simulink model "ctrlSys"  (R2025b)
settings: Solver=ode14x  StartTime=0.0  StopTime=70  FixedStep=Ts_local  RelTol=1e-4
model workspace (MAT data in the model file):
  CtrlChoice = "GPC"
values from neighbouring files (symbols this model uses):
  Ts_ctrl = 0.1    [ctrlSys.sldd]
  u_b = 0.5864    [ctrlSys.sldd]
libraries: slpidlib x1
settings Model: DataDictionary=ctrlSys.sldd  SimulationMode=accelerator  Creator=LYG  LastModifiedBy=LYG
settings SolverCC: ZeroCrossControl=DisableAll

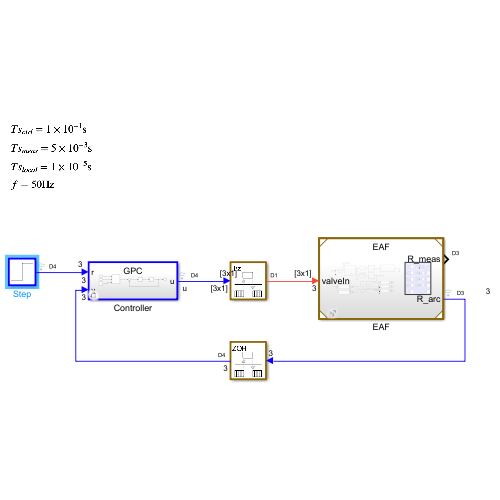
[thumbnail: Simulink's stored preview of the top-level diagram]
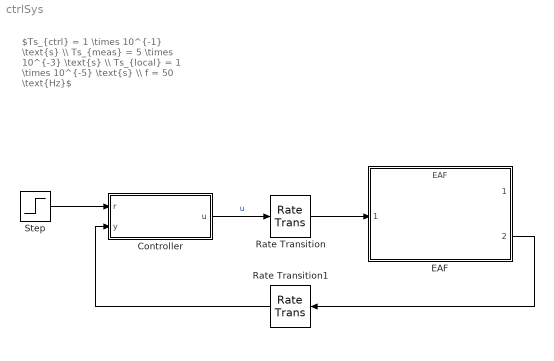
== system ctrlSys ==
  note: $Ts_{ctrl} = 1 \times 10^{-1} \text{s} \\ Ts_{meas} = 5 \times 10^{-3} \text{s} \\ Ts_{local} = 1 \times 10^{-5} \text{s} \\ f = 50 \text{Hz}$
  Controller : Subsystem  Variant=on
  EAF : ModelReference  ModelNameDialog=EAF.slx  SimulationMode=Normal  ModelReferenceVersion=1.75
  Rate Transition : RateTransition  InitialCondition=u_b  OutPortSampleTime=Ts_local
  Rate Transition1 : RateTransition  OutPortSampleTime=Ts_ctrl
  Step : Step  Time=20  Before=[0.025 0.01 0.075]  After=[0.025 0.02 0.075]  SampleTime=Ts_ctrl
  wires:
  Controller/1(u) -> Rate Transition/1  "u"
  Rate Transition/1 -> EAF/1
  EAF/2 -> Rate Transition1/1
  Step/1 -> Controller/1(r)
  Rate Transition1/1 -> Controller/2(y)

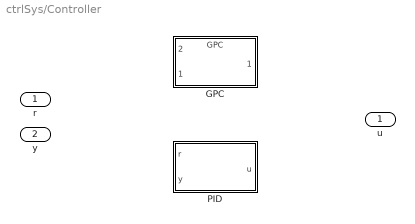
== system ctrlSys/Controller ==
  r : Inport
  y : Inport  Port=2
  GPC : ModelReference  ModelNameDialog=GPC.slx  SimulationMode=Normal  VariantControl="CtrlChoice == \"GPC\""  ModelReferenceVersion=1.202
      settings: PortSchema="{\"entries\":[{\"content\":{\"sides\":[{\"content\":{\"connectorIds\":[\"In2\",\"In1\"]},\"type\":\"ConnectorPlacement.EquallySpacedRectSide\",\"uuid\":\"c107f1c2-3547-45d9-8105-1f531098cad9\"},{\"content\":{\"connectorIds\":[\"Out1\"],\"side\":\"RIGHT\"},\"type\":\"ConnectorPlacement.EquallySpacedRectSide\",\"uuid\":\"edcbd001-1fd9-492d-b847-8c21cda39726\"},{\"content\":{\"side\":\"TOP\"},\"type\":\"ConnectorPlacement.EquallySpacedRectSide\",\"uuid\":\"231ba3de-6bd5-4532-a826-5d19b482de4e\"}]},\"type\":\"ConnectorPlacement.EquallySpacedConnector\",\"uuid\":\"eca704b6-0f9b-48e0-aad6-a98053cf6fe0\"}],\"packageUris\":[\"http://schema.mathworks.com/mf0/Connector/R2020b\"],\"version\":\"1.0\"}"
  PID : Subsystem  VariantControl="CtrlChoice == \"PID\""
  u : Outport

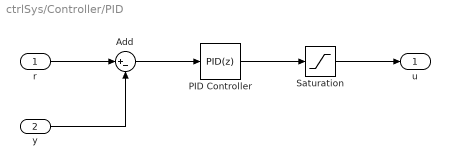
== system ctrlSys/Controller/PID ==
  r : Inport
  y : Inport  Port=2
  Add : Sum  Inputs=|+-
  PID Controller : slpidlib/PID Controller  Controller=PID  Form=Parallel  TimeDomain=Discrete-time  UseExternalTs=off  SampleTime=Ts_ctrl  IntegratorMethod=Forward Euler  FilterMethod=Forward Euler  ControllerParametersSource=internal  P=120  I=40  UseKiTs=off  D=0  UseExternalDerivativeSource=off  N=100  UseFilter=on  TunerSelectOption=Transfer Function Based (PID Tuner App)  InitialConditionSource=internal  InitialConditionForIntegrator=0  InitialConditionForFilter=0  DifferentiatorICPrevScaledInput=0  ExternalReset=none  TrackingMode=off  Kt=1  LimitOutput=off  SatLimitsSource=internal  UpperSaturationLimit=inf  LowerSaturationLimit=-inf  LinearizeAsGain=on  AntiWindupMode=none  Kb=1  LimitIntegrator=off  UpperIntegratorSaturationLimit=inf  LowerIntegratorSaturationLimit=-inf  POutMin=[]  POutMax=[]  IOutMin=[]  IOutMax=[]  DOutMin=[]  DOutMax=[]  NOutMin=[]  NOutMax=[]  SumOutMin=[]  SumOutMax=[]  SaturationOutMin=[]  SaturationOutMax=[]  PParamMin=[]  PParamMax=[]  IParamMin=[]  IParamMax=[]  DParamMin=[]  DParamMax=[]  NParamMin=[]  NParamMax=[]  KbParamMin=[]  KbParamMax=[]  KtParamMin=[]  KtParamMax=[]  KbOutMin=[]  KbOutMax=[]  KtOutMin=[]  KtOutMax=[]  IntegratorOutMin=[]  IntegratorOutMax=[]  FilterOutMin=[]  FilterOutMax=[]  SumI1OutMin=[]  SumI1OutMax=[]  SumI2OutMin=[]  SumI2OutMax=[]  SumI3OutMin=[]  SumI3OutMax=[]  SumI4OutMin=[]  SumI4OutMax=[]  SumDOutMin=[]  SumDOutMax=[]  DifferentiatorOutMin=[]  DifferentiatorOutMax=[]  FilterDiffOutCoefMin=[]  FilterDiffOutCoefMax=[]  ReciprocalOutMin=[]  ReciprocalOutMax=[]  SumDenOutMin=[]  SumDenOutMax=[]  SumNumOutMin=[]  SumNumOutMax=[]  DivideOutMin=[]  DivideOutMax=[]  UdiffTsProdOutMin=[]  UdiffTsProdOutMax=[]  NTsProdOutMin=[]  NTsProdOutMax=[]  UintegralTsProdOutMin=[]  UintegralTsProdOutMax=[]  UngainTsProdOutMin=[]  UngainTsProdOutMax=[]  ClampingZeroOutDataTypeStr=Inherit: Inherit via back propagation  ClampingZeroOutMin=[]  ClampingZeroOutMax=[]  FilterDenConstantOutDataTypeStr=Inherit: Inherit via back propagation  FilterDenConstantOutMin=[]  FilterDenConstantOutMax=[]  PCopyOutDataTypeStr=Inherit: Inherit via back propagation  PCopyOutMin=[]  PCopyOutMax=[]  NCopyOutDataTypeStr=Inherit: Inherit via back propagation  NCopyOutMin=[]  NCopyOutMax=[]  IntegratorContinuousStateAttributes=''  IntegratorStateMustResolveToSignalObject=off  IntegratorRTWStateStorageClass=Auto  FilterContinuousStateAttributes=''  FilterStateMustResolveToSignalObject=off  FilterRTWStateStorageClass=Auto  ParallelPVariant=InternalParameters  IdealPVariant=Disabled  IVariant=InternalParameters  DVariant=InternalParameters  IntegratorVariant=Discrete  SatVariant=Disabled  AWVariant=Passthrough  PCopyVariant=Disabled  TRVariant=Disabled  FdbkBlocksVariant=Forward  IdealPFdbkVariant=Disabled  SatFdbkVariant=Disabled  DerivativeFilterVariant=ForwardEulerFilter  NVariant=InternalParameters  NCopyVariant=Disabled  FilterICVariant=InternalICsFilter  IntegratorICVariant=InternalICs  ExternalResetVariant=Disabled  TRSumVariant=Passthrough  SumFdbkVariant=Disabled  SumVariant=Sum_PID  TsampFilterVariant=InternalTs  TsampNgainVariant=Passthrough  TsampIntegralVariant=Disabled_SignalSpec  ExternalSaturationOutDataTypeStr=Inherit: Same as second input  DerivativeSourceVariant=ErrorSignal  PreIntVariant=InternalPreInt
  Saturation : Saturate  UpperLimit=1.12  LowerLimit=-1.08
  u : Outport
  wires:
  r/1 -> Add/1
  Add/1 -> PID Controller/1
  y/1 -> Add/2
  Saturation/1 -> u/1
  PID Controller/1 -> Saturation/1
